simulink model "DCmotorAItuning"  (R2025b)
settings: Solver=VariableStepAuto  StartTime=0.0  StopTime=2  RelTol=1e-3
values from neighbouring files (symbols this model uses):
  A11 = base_A11 * (1 + plant_variation_percent * (2*rand - 1))    [make_training_case.m]
  A12 = base_A12 * (1 + plant_variation_percent * (2*rand - 1))    [make_training_case.m]
  A21 = base_A21 * (1 + plant_variation_percent * (2*rand - 1))    [make_training_case.m]
  A22 = base_A22 * (1 + plant_variation_percent * (2*rand - 1))    [make_training_case.m]
  B1 = base_B1  * (1 + plant_variation_percent * (2*rand - 1))    [make_training_case.m]
  Kd = 0.8951    [make_training_case.m]    (also in run_pid_search.m)
  Ki = 57.4007    [make_training_case.m]    (also in run_pid_search.m)
  Kp = 15.0380    (= 15.038)    [run_pid_search.m]
  Nf = 1159.8    [make_training_case.m]    (also in pid_search_results.mat; run_pid_search.m)
  step_amp = min_step_amp + (max_step_amp - min_step_amp) * rand    [make_training_case.m]
libraries: slpidlib x1
settings Model: Creator=karno  LastModifiedBy=karno

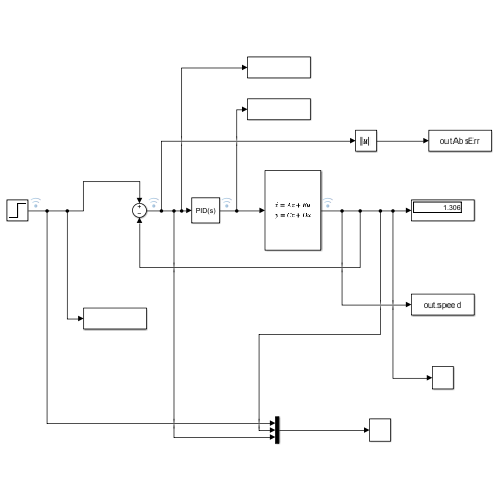
[thumbnail: Simulink's stored preview of the top-level diagram]
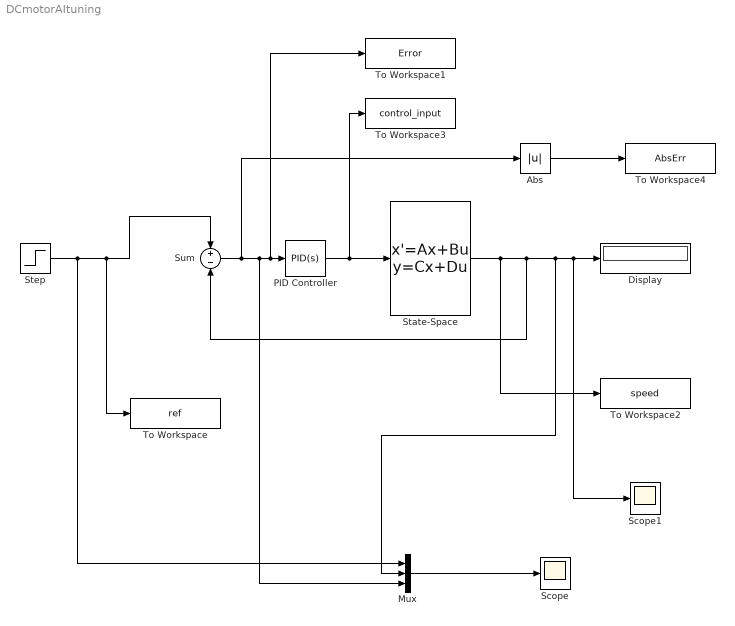
== system DCmotorAItuning ==
  Abs : Abs  SaturateOnIntegerOverflow=off
  Display : Display
  Mux : Mux  Inputs=3
  PID Controller : slpidlib/PID Controller  Controller=PID  Form=Parallel  TimeDomain=Continuous-time  UseExternalTs=off  SampleTime=-1  IntegratorMethod=Forward Euler  FilterMethod=Forward Euler  ControllerParametersSource=internal  P=Kp  I=Ki  UseKiTs=off  D=Kd  UseExternalDerivativeSource=off  N=Nf  UseFilter=on  TunerSelectOption=Transfer Function Based (PID Tuner App)  InitialConditionSource=internal  InitialConditionForIntegrator=0  InitialConditionForFilter=0  DifferentiatorICPrevScaledInput=0  ExternalReset=none  TrackingMode=off  Kt=1  LimitOutput=off  SatLimitsSource=internal  UpperSaturationLimit=inf  LowerSaturationLimit=-inf  LinearizeAsGain=on  AntiWindupMode=none  Kb=1  LimitIntegrator=off  UpperIntegratorSaturationLimit=inf  LowerIntegratorSaturationLimit=-inf  POutMin=[]  POutMax=[]  IOutMin=[]  IOutMax=[]  DOutMin=[]  DOutMax=[]  NOutMin=[]  NOutMax=[]  SumOutMin=[]  SumOutMax=[]  SaturationOutMin=[]  SaturationOutMax=[]  PParamMin=[]  PParamMax=[]  IParamMin=[]  IParamMax=[]  DParamMin=[]  DParamMax=[]  NParamMin=[]  NParamMax=[]  KbParamMin=[]  KbParamMax=[]  KtParamMin=[]  KtParamMax=[]  KbOutMin=[]  KbOutMax=[]  KtOutMin=[]  KtOutMax=[]  IntegratorOutMin=[]  IntegratorOutMax=[]  FilterOutMin=[]  FilterOutMax=[]  SumI1OutMin=[]  SumI1OutMax=[]  SumI2OutMin=[]  SumI2OutMax=[]  SumI3OutMin=[]  SumI3OutMax=[]  SumI4OutMin=[]  SumI4OutMax=[]  SumDOutMin=[]  SumDOutMax=[]  DifferentiatorOutMin=[]  DifferentiatorOutMax=[]  FilterDiffOutCoefMin=[]  FilterDiffOutCoefMax=[]  ReciprocalOutMin=[]  ReciprocalOutMax=[]  SumDenOutMin=[]  SumDenOutMax=[]  SumNumOutMin=[]  SumNumOutMax=[]  DivideOutMin=[]  DivideOutMax=[]  UdiffTsProdOutMin=[]  UdiffTsProdOutMax=[]  NTsProdOutMin=[]  NTsProdOutMax=[]  UintegralTsProdOutMin=[]  UintegralTsProdOutMax=[]  UngainTsProdOutMin=[]  UngainTsProdOutMax=[]  ClampingZeroOutDataTypeStr=Inherit: Inherit via back propagation  ClampingZeroOutMin=[]  ClampingZeroOutMax=[]  FilterDenConstantOutDataTypeStr=Inherit: Inherit via back propagation  FilterDenConstantOutMin=[]  FilterDenConstantOutMax=[]  PCopyOutDataTypeStr=Inherit: Inherit via back propagation  PCopyOutMin=[]  PCopyOutMax=[]  NCopyOutDataTypeStr=Inherit: Inherit via back propagation  NCopyOutMin=[]  NCopyOutMax=[]  IntegratorContinuousStateAttributes=''  IntegratorStateMustResolveToSignalObject=off  IntegratorRTWStateStorageClass=Auto  FilterContinuousStateAttributes=''  FilterStateMustResolveToSignalObject=off  FilterRTWStateStorageClass=Auto  ParallelPVariant=InternalParameters  IdealPVariant=Disabled  IVariant=InternalParameters  DVariant=InternalParameters  IntegratorVariant=Continuous  SatVariant=Disabled  AWVariant=Passthrough  PCopyVariant=Disabled  TRVariant=Disabled  FdbkBlocksVariant=Forward  IdealPFdbkVariant=Disabled  SatFdbkVariant=Disabled  DerivativeFilterVariant=ContFilter  NVariant=InternalParameters  NCopyVariant=Disabled  FilterICVariant=InternalICsFilter  IntegratorICVariant=InternalICs  ExternalResetVariant=Disabled  TRSumVariant=Passthrough  SumFdbkVariant=Disabled  SumVariant=Sum_PID  TsampFilterVariant=InternalTs  TsampNgainVariant=Passthrough  TsampIntegralVariant=Disabled_SignalSpec  ExternalSaturationOutDataTypeStr=Inherit: Same as second input  DerivativeSourceVariant=ErrorSignal  PreIntVariant=InternalPreInt
  Scope : Scope
      settings: ActiveDisplayYMinimum=-0.23489684025241708  ActiveDisplayYMaximum=1.2483995046105596
  Scope1 : Scope
      settings: ActiveDisplayYMinimum=-0.48706785125124352  ActiveDisplayYMaximum=1.54368039970724
  State-Space : StateSpace  A=[A11 A12; A21 A22]  B=[B1; 0]  C=[0 1]  D=0  InitialCondition=[0;0]
  Step : Step  Time=0  After=step_amp  SampleTime=0
  Sum : Sum  Inputs=+-
  To Workspace : ToWorkspace  VariableName=ref  SampleTime=-1
  To Workspace1 : ToWorkspace  VariableName=Error  SampleTime=-1
  To Workspace2 : ToWorkspace  VariableName=speed  SampleTime=-1
  To Workspace3 : ToWorkspace  VariableName=control_input  SampleTime=-1
  To Workspace4 : ToWorkspace  VariableName=AbsErr  SampleTime=-1
  wires:
  Step/1 -> Sum/1, To Workspace/1, Mux/1
  Sum/1 -> Abs/1, Mux/3, To Workspace1/1, PID Controller/1
  PID Controller/1 -> To Workspace3/1, State-Space/1
  State-Space/1 -> To Workspace2/1, Mux/2, Scope1/1, Display/1, Sum/2
  Mux/1 -> Scope/1
  Abs/1 -> To Workspace4/1
